simulink model "PhotodetectorModel1"  (R2020b)
settings: Solver=VariableStepAuto  StartTime=0.0  StopTime=0.5  RelTol=1e-3
model workspace (MAT data in the model file):
  A1 = 0.25
  A2 = 0.25
  C1 = 1.8
  C2 = 1.8
  Id1 = 0.1
  Id2 = 0.1
  Ip1 = 0.52
  Ip2 = 0.52
  Rload1 = 50
  Rload2 = 50
  Rs1 = 10
  Rs2 = 10
  Rshunt1 = 1000
  Rshunt2 = 1000
  StepF = 0.52
  Vf1 = 1.3
  Vf2 = 1.3
libraries: fl_lib x12, nesl_utility x5, ee_lib x3, simulink x1
settings Model: OrderedModelArguments=off  Creator=mic_b  LastModifiedBy=bolic
settings DataIOCC: ReturnWorkspaceOutputsName=SDOSimTest_Log
settings SFSimCC: CustomCodeUndefinedFunction=UseInterfaceOnly

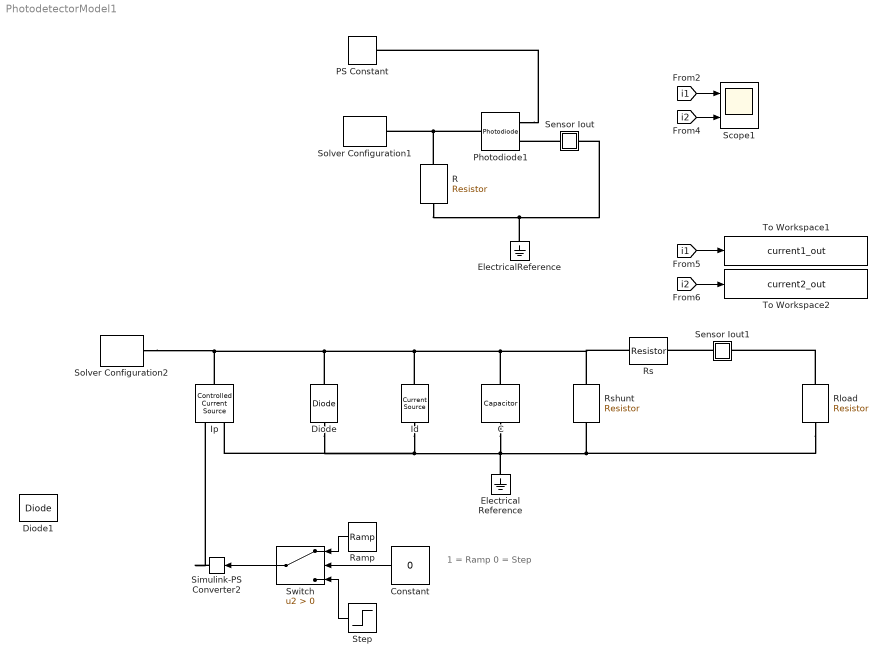
== system PhotodetectorModel1 ==
  note: 1 = Ramp
      | 0 = Step
  C : fl_lib/Electrical/Electrical Elements/Capacitor  c=3.5 pF  r=1e-6 Ohm  g=0 1/Ohm  i_specify=off  i_priority=None  i=0 A  i_nominal_specify=off  i_nominal_unit=A  i_nominal_value=1  v_specify=off  v_priority=None  v=0 V  v_nominal_specify=off  v_nominal_unit=V  v_nominal_value=1  vc_specify=off  vc_priority=High  vc=0 V  vc_nominal_specify=off  vc_nominal_unit=V  vc_nominal_value=1
  Constant : Constant  Value=0  VectorParams1D=off  SampleTime=-1
  Diode : fl_lib/Electrical/Electrical Elements/Diode  Vf=1.3 V  Ron=0.3 Ohm  Goff=1e-8 1/Ohm  i_specify=off  i_priority=None  i=0 A  i_nominal_specify=off  i_nominal_unit=A  i_nominal_value=1  v_specify=off  v_priority=None  v=0 V  v_nominal_specify=off  v_nominal_unit=V  v_nominal_value=1
  Diode1 : ee_lib/Semiconductors & Converters/Diode  ModelType=ee.enum.diode.modelType.exponential  IfMat=[.07, .12, .19, 1.75, 4.24, 7.32, 11.2; .16, .3, .72, 2.14, 4.02, 6.35, 9.12] A  TjVec=[25, 125] degC  VfVec=[.5, .7, .9, 1.3, 1.7, 2.1, 2.5] V  Vf=0.6 V  Ron=0.3 Ohm  Goff=1e-8 S  prmExp=ee.enum.diode.expParam.useIVIs  I12=[.0137, .545] A  V12=[.6, .7] V  IS=0.2 nA  ec=1  I1=0.0137 A  V1=0.6 V  RS=0 Ohm  Tmeas=25 degC  N_series=1  N_parallel=1  Rz=0.3 Ohm  BV=inf V  C_param=ee.enum.diode.capParam.fixed  CJ=5 pF  CJ0=5 pF  VJ=1 V  Mgrad=0.5  Vvec=[.1, 10, 100] V  Cvec=[3.5, 1, .4] pF  FC=0.5  Q_param=ee.enum.diode.recoveryParam.off  iRM=-7.15 A  iF=4 A  didt=-750 A/us  trr_factor=3  trr=115 ns  Qrr=1500 s*uA  TT=50 ns  tau=100 ns  T_param=ee.enum.diode.temperatureParam.off  IS_T2=1.25e-7 A  I1_T2=0.245 A  V1_T2=0.5 V  Tmeas2=125 degC  EG_param=ee.enum.diode.egapParam.material_si  EG=1.11 eV  XTI_param=ee.enum.diode.xtiParam.pn  XTI=3  dBVdT=0 V/K  Tdevice=25 degC  i_specify=off  i_priority=None  i=0 A  i_nominal_specify=off  i_nominal_unit=A  i_nominal_value=1  v_specify=off  v_priority=None  v=0 V  v_nominal_specify=off  v_nominal_unit=V  v_nominal_value=1  i_capacitor_specify=off  i_capacitor_priority=None  i_capacitor=0 A  i_capacitor_nominal_specify=off  i_capacitor_nominal_unit=A  i_capacitor_nominal_value=1  v_capacitor_specify=off  v_capacitor_priority=None  v_capacitor=0 V  v_capacitor_nominal_specify=off  v_capacitor_nominal_unit=V  v_capacitor_nominal_value=1  power_dissipated_specify=off  power_dissipated_priority=None  power_dissipated=0 W  power_dissipated_nominal_specify=off  power_dissipated_nominal_unit=W  power_dissipated_nominal_value=1  thermal_network_parameterization=ee.enum.thermalNetworkTopology.cauer  Rth=[0, 10] K/W  Rth_Foster=[4, 6] K/W  thermal_mass_parameterization=ee.enum.thermalNetwork.timeconstant  thermal_mass=[0, 1] J/K  thermal_mass_Foster=[1.5, 3] J/K  thermal_time_constant=[0, 10] s  thermal_time_constant_Foster=[6, 18] s  thermal_mass_initial_temperatures=[25, 25] degC
  Electrical Reference : fl_lib/Electrical/Electrical Elements/Electrical Reference
  ElectricalReference : fl_lib/Electrical/Electrical Elements/Electrical Reference
  Id : ee_lib/Sources/Current Source  dc_current=0.2 nA  ac_current=0 A  ac_shift=0 rad  ac_frequency=60 Hz  noise_mode=0  PSD=0 A^2/Hz  repeatability=1  auto_seed=913116633  user_seed=0  sample_time=1e-3 s  i_specify=off  i_priority=None  i=0 A  i_nominal_specify=off  i_nominal_unit=A  i_nominal_value=1  v_specify=off  v_priority=None  v=0 V  v_nominal_specify=off  v_nominal_unit=V  v_nominal_value=1
      settings: SourceProductBaseCode=PS
  Ip : fl_lib/Electrical/Electrical Sources/Controlled Current Source
  "PS Constant " : fl_lib/Physical Signals/Sources/PS Constant  constant=0.001/0.25 W/mm^2
  Photodiode1 : ee_lib/Sensors & Transducers/Photodiode  prmFlux=2  Imeas=25 uA  FluxD=5 W/m^2  G=0.52 mm^2*A/W  prmExp=1  I2=0.1 A  V2=1.3 V  IS=0.2 nA  ec=3  RS=0.1 Ohm  Tmeas=23 degC  C_param=1  CJ=1.8 pF  CJ0=60 pF  VJ=1 V  Mgrad=0.5  Vvec=[.1, 10, 100] V  Cvec=[45, 3, 6] pF  FC=0.5  T_param=1  IS_T2=2.5e-7 A  I1_T2=0.07 A  V1_T2=1.3 V  Tmeas2=125 degC  EG_param=1  EG=1.11 eV  XTI_param=1  XTI=3  Tdevice=25 degC  i_capacitor_specify=off  i_capacitor_priority=High  i_capacitor=0 A  i_capacitor_nominal_specify=off  i_capacitor_nominal_unit=A  i_capacitor_nominal_value=1  v_capacitor_specify=off  v_capacitor_priority=None  v_capacitor=0 V  v_capacitor_nominal_specify=off  v_capacitor_nominal_unit=V  v_capacitor_nominal_value=1  thermal_network_parameterization=ee.enum.thermalNetworkTopology.cauer  Rth=[0, 10] K/W  Rth_Foster=[4, 6] K/W  thermal_mass_parameterization=1  thermal_mass=[0, 1] J/K  thermal_mass_Foster=[1.5, 3] J/K  thermal_time_constant=[0, 10] s  thermal_time_constant_Foster=[6, 18] s  thermal_mass_initial_temperatures=[25, 25] degC
      settings: SourceProductBaseCode=PS  InternalSimscapePortConfiguration="{\"Bottom\":[],\"Left\":[{\"id\":\"W\",\"label\":\"W\",\"type\":\"input\"},{\"id\":\"p\",\"label\":\"\",\"type\":\"foundation.electrical.electrical\"}],\"Right\":[{\"id\":\"n\",\"label\":\"\",\"type\":\"foundation.electrical.electrical\"}],\"Top\":[]}"
  R : fl_lib/Electrical/Electrical Elements/Resistor  R=60 Ohm  i_specify=off  i_priority=None  i=0 A  i_nominal_specify=off  i_nominal_unit=A  i_nominal_value=1  v_specify=off  v_priority=None  v=0 V  v_nominal_specify=off  v_nominal_unit=V  v_nominal_value=1
  "Ramp " : simulink/Sources/Ramp  slope=0.52  start=0  InitialOutput=0
  Rload : fl_lib/Electrical/Electrical Elements/Resistor  R=50 Ohm  i_specify=off  i_priority=None  i=0 A  i_nominal_specify=off  i_nominal_unit=A  i_nominal_value=1  v_specify=off  v_priority=None  v=0 V  v_nominal_specify=off  v_nominal_unit=V  v_nominal_value=1
  Rs : fl_lib/Electrical/Electrical Elements/Resistor  R=10 Ohm  i_specify=off  i_priority=None  i=0 A  i_nominal_specify=off  i_nominal_unit=A  i_nominal_value=1  v_specify=off  v_priority=None  v=0 V  v_nominal_specify=off  v_nominal_unit=V  v_nominal_value=1
  Rshunt : fl_lib/Electrical/Electrical Elements/Resistor  R=500 MOhm  i_specify=off  i_priority=None  i=0 A  i_nominal_specify=off  i_nominal_unit=A  i_nominal_value=1  v_specify=off  v_priority=None  v=0 V  v_nominal_specify=off  v_nominal_unit=V  v_nominal_value=1
  Scope1 : Scope  NumInputPorts=2
  Sensor Iout : Subsystem
      mask Display: disp('i')
  Sensor Iout1 : Subsystem
      mask Display: disp('i')
  "Simulink-PS Converter2 " : nesl_utility/Simulink-PS Converter  PhysicalDomain=network_engine_domain  SubClassName=ps_input  LeftPortType=input  RightPortType=output  PseudoPeriodic=off  Frequencies=[]  NoiseDistribution=none  NoiseParameters=[]  Unit=1  AffineConversion=off  FilteringAndDerivatives=provide  SimscapeFilterOrder=1  InputFilterTimeConstant=0.001  UdotUserProvided=0
  "Solver Configuration1 " : nesl_utility/Solver Configuration  PhysicalDomain=network_engine_domain  SubClassName=solver  LeftPortType=input  RightPortType=generic  Tones=[]  Harmonics=[]  SimulateNoise=off  Profile=off  UseLocalSampling=off  EnableSwitchedLinearOptims=on  FrequencyDomain=off  UseCCode=off  RelTol=0.001  AbsTol=1e-06  MinStep=1e-09  ToWorkspace=off  RevertToSquareIcSolve=off  NumHomotopyIterations=100  PhasorMode=off  PhasorModeNumHarmonics=1  DoDC=off  ResidualTolerance=1e-09  UseLocalSolver=off  LocalSolverChoice=NE_BACKWARD_EULER_ADVANCER  LocalSolverSampleTime=0.001  DoFixedCost=off  MaxNonlinIter=3  MaxModeIter=2  ComputeImpulses=off  ImpulseIterations=2  LinearAlgebra=auto  EquationFormulation=NE_TIME_EF  DelaysMemoryBudget=1024  AutomaticFiltering=on  FilteringTimeConstant=0.001  PartitionStorageMethod=AS_NEEDED  PartitionMemoryBudget=1024  PartitionMethod=ROBUST
  "Solver Configuration2 " : nesl_utility/Solver Configuration  PhysicalDomain=network_engine_domain  SubClassName=solver  LeftPortType=input  RightPortType=generic  Tones=[]  Harmonics=[]  SimulateNoise=off  Profile=off  UseLocalSampling=off  EnableSwitchedLinearOptims=on  FrequencyDomain=off  UseCCode=off  RelTol=0.001  AbsTol=1e-06  MinStep=1e-09  ToWorkspace=off  RevertToSquareIcSolve=off  NumHomotopyIterations=100  PhasorMode=off  PhasorModeNumHarmonics=1  DoDC=off  ResidualTolerance=1e-09  UseLocalSolver=off  LocalSolverChoice=NE_BACKWARD_EULER_ADVANCER  LocalSolverSampleTime=0.001  DoFixedCost=off  MaxNonlinIter=3  MaxModeIter=2  ComputeImpulses=off  ImpulseIterations=2  LinearAlgebra=auto  EquationFormulation=NE_TIME_EF  DelaysMemoryBudget=1024  AutomaticFiltering=on  FilteringTimeConstant=0.001  PartitionStorageMethod=AS_NEEDED  PartitionMemoryBudget=1024  PartitionMethod=ROBUST
  Step : Step  Time=0  After=0.00013  SampleTime=0
  "Switch " : Switch  Criteria=u2 > Threshold
  To Workspace1 : ToWorkspace  VariableName=current1_out  SaveFormat=Timeseries  SampleTime=-1
  To Workspace2 : ToWorkspace  VariableName=current2_out  SaveFormat=Timeseries  SampleTime=-1
  wires:
  Step/1 -> "Switch "/3
  "Switch "/1 -> "Simulink-PS Converter2 "/1
  "Ramp "/1 -> "Switch "/1
  Constant/1 -> "Switch "/2
  [i1] -> Scope1/1
  [i2] -> Scope1/2
  [i1] -> To Workspace1/1
  [i2] -> To Workspace2/1
  connections:
  Diode/LConn1 -- Rshunt/LConn1 -- Rs/LConn1 -- C/LConn1 -- Id/LConn1 -- Ip/LConn1 -- "Solver Configuration2 "/RConn1
  Rload/LConn1 -- Sensor Iout1/LConn1
  Rload/RConn1 -- C/RConn1 -- Electrical Reference/LConn1 -- Diode/RConn1 -- Ip/RConn2 -- Id/RConn1 -- Rshunt/RConn1
  Sensor Iout1/RConn1 -- Rs/RConn1
  ElectricalReference/LConn1 -- Sensor Iout/LConn1 -- R/RConn1
  Sensor Iout/RConn1 -- Photodiode1/LConn2
  Photodiode1/LConn1 -- "PS Constant "/RConn1
  Photodiode1/RConn1 -- R/LConn1 -- "Solver Configuration1 "/RConn1
  "Simulink-PS Converter2 "/RConn1 -- Ip/RConn1

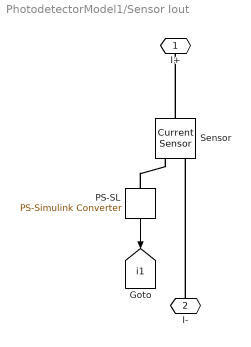
== system PhotodetectorModel1/Sensor Iout ==
  PS-SL : nesl_utility/PS-Simulink Converter  PhysicalDomain=network_engine_domain  SubClassName=ps_output  LeftPortType=input  RightPortType=output  PseudoPeriodic=off  Frequencies=[]  Unit=1  AffineConversion=off
  Sensor : fl_lib/Electrical/Electrical Sensors/Current Sensor
      settings: SourceProductName=Foundation Library
  I+ : PMIOPort  Side=Right
  I- : PMIOPort  Port=2  Side=Left
  tag scope: i1=global
  wires:
  PS-SL/1 -> [i1]
  connections:
  PS-SL/LConn1 -- Sensor/RConn1
  Sensor/LConn1 -- I+/RConn1
  I-/RConn1 -- Sensor/RConn2

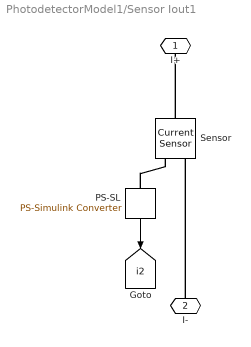
== system PhotodetectorModel1/Sensor Iout1 ==
  PS-SL : nesl_utility/PS-Simulink Converter  PhysicalDomain=network_engine_domain  SubClassName=ps_output  LeftPortType=input  RightPortType=output  PseudoPeriodic=off  Frequencies=[]  Unit=1  AffineConversion=off
  Sensor : fl_lib/Electrical/Electrical Sensors/Current Sensor
      settings: SourceProductName=Foundation Library
  I+ : PMIOPort  Side=Right
  I- : PMIOPort  Port=2  Side=Left
  tag scope: i2=global
  wires:
  PS-SL/1 -> [i2]
  connections:
  PS-SL/LConn1 -- Sensor/RConn1
  Sensor/LConn1 -- I+/RConn1
  I-/RConn1 -- Sensor/RConn2
